simulink model "LBR7_Single_JointComputedTorque"  (R2017b)
settings: Solver=FixedStepAuto  StartTime=0.0  StopTime=12  FixedStep=0.01  RelTol=1e-3
PreLoadFcn:
  | Preload
values from neighbouring files (symbols this model uses):
  cor_gain = -1    [Preload.m]
  joint1_gain = 1    [Preload.m]    (also in PreloadTest.m)
  joint1_initial_deg = 0    [Preload.m]    (also in PreloadTest.m = 25)
  joint2_gain = 1    [Preload.m]    (also in PreloadTest.m)
  joint2_initial_deg = 0    [Preload.m]    (also in PreloadTest.m = 70)
  joint3_gain = 1    [Preload.m]    (also in PreloadTest.m)
  joint3_initial_deg = -25    [Preload.m]    (also in PreloadTest.m = 60)
  joint4_gain = 1    [Preload.m]    (also in PreloadTest.m)
  joint4_initial_deg = 90    [Preload.m]    (also in PreloadTest.m = 20)
  joint5_gain = 1    [Preload.m]    (also in PreloadTest.m)
  joint5_initial_deg = 0    [Preload.m]    (also in PreloadTest.m = 22)
  joint6_gain = 1    [Preload.m]    (also in PreloadTest.m)
  joint6_initial_deg = 90    [Preload.m]    (also in PreloadTest.m = 60)
  joint7_gain = 1    [Preload.m]    (also in PreloadTest.m)
  joint7_initial_deg = 0    [Preload.m]    (also in PreloadTest.m = 30)
  kuk = SerialLink(L)    [Preload.m]    (also in PreloadTest.m)
undefined symbols (not defined in the file or in its folder): cory, gravy, inert, X, Y, Z
libraries: sm_lib x77, nesl_utility x30
(part 1 of 3)
settings Model: Creator=jrv  LastModifiedBy=mkiri

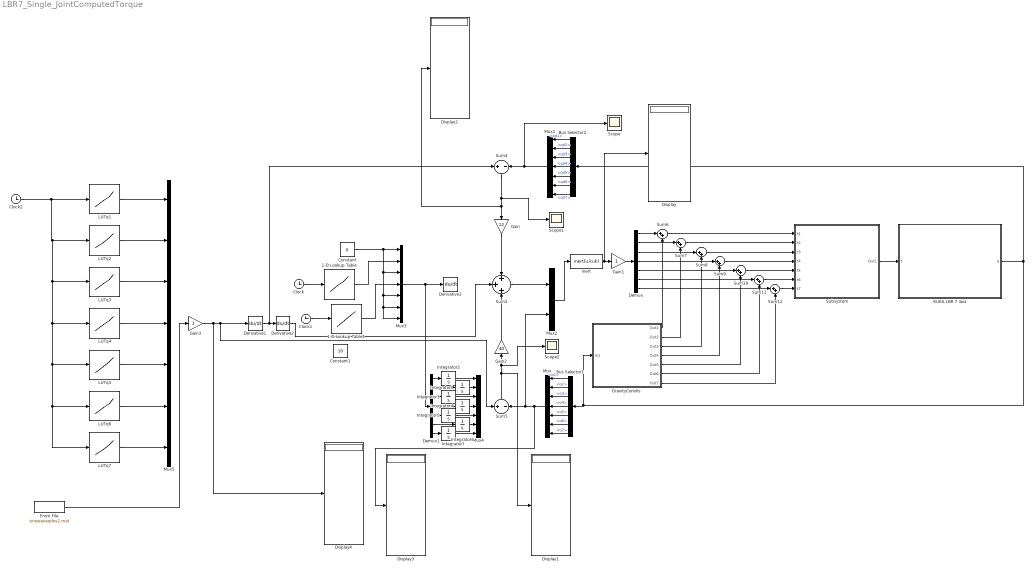
== system LBR7_Single_JointComputedTorque ==
  1-D Lookup Table : Lookup_n-D  NumberOfTableDimensions=1  BreakpointsForDimension1=[0 3 6]  Table=[0 -0.05 -0.1]  ExtrapMethod=Clip  UseLastTableValue=on  InternalRulePriority=Speed  RndMeth=Simplest  InputSameDT=on
  1-D Lookup Table1 : Lookup_n-D  NumberOfTableDimensions=1  BreakpointsForDimension1=[0 3 6]  Table=[0 -0.05 -0.1]  ExtrapMethod=Clip  UseLastTableValue=on  InternalRulePriority=Speed  RndMeth=Simplest  InputSameDT=on
  Bus Selector1 : BusSelector  OutputSignals=q1,q2,q3,q4,q5,q6,q7
  Bus Selector2 : BusSelector  OutputSignals=qd1,qd2,qd3,qd4,qd5,qd6,qd7
  Clock : Clock
  Clock1 : Clock
  Clock2 : Clock
  Constant : Constant  Value=0
  Constant1 : Constant  Value=10
  Demux : Demux  Outputs=7
  Demux1 : Demux  Outputs=7
  Derivative1 : Derivative
  Derivative2 : Derivative
  Derivative3 : Derivative
  Display{,1..4} (5 alike) : Display
  From File : FromFile  FileName=sinewaveqdes2.mat  SampleTime=0
  Gain : Gain  Gain=12
  Gain1 : Gain
  Gain2 : Gain  Gain=40
  Gain3 : Gain
  GravityCoriolis : Subsystem
  Integrator1 : Integrator  InitialCondition=joint2_initial_deg*pi/180
  Integrator2 : Integrator  InitialCondition=joint1_initial_deg*pi/180
  Integrator3 : Integrator  InitialCondition=joint3_initial_deg*pi/180
  Integrator4 : Integrator  InitialCondition=joint4_initial_deg*pi/180
  Integrator5 : Integrator  InitialCondition=joint5_initial_deg*pi/180
  Integrator6 : Integrator  InitialCondition=joint6_initial_deg*pi/180
  Integrator7 : Integrator  InitialCondition=joint7_initial_deg*pi/180
  KUKA LBR 7 iiwa : Subsystem
  LUTq1 : Lookup_n-D  NumberOfTableDimensions=1  BreakpointsForDimension1=|  Table=|  ExtrapMethod=Clip  UseLastTableValue=on  InternalRulePriority=Speed  RndMeth=Simplest  InputSameDT=on
      | [0
      | 0.1
      | 0.2
      | 0.3
      | 0.4
      | 0.5
      | 0.6
      | 0.7
      | 0.8
      | 0.9
      | 1
      | 1.1
      | 1.2
      | 1.3
      | 1.4
      | 1.5
      | 1.6
      | 1.7
      | 1.8
      | 1.9
      | 2
      | 2.1
      | 2.2
      | 2.3
      | 2.4
      | 2.5
      | 2.6
      | 2.7
      | 2.8
      | 2.9
      | 3
      | 3.1
      | 3.2
      | 3.3
      | 3.4
      | 3.5
      | 3.6
      | 3.7
      | 3.8
      | 3.9
      | 4
      | 4.1
      | 4.2
      | 4.3
      | 4.4
      | 4.5
      | 4.6
      | 4.7
      | 4.8
      | 4.9
      | 5
      | 5.1
      | 5.2
      | 5.3
      | 5.4
      | 5.5
      | 5.6
      | 5.7
      | 5.8
      | 5.9
      | 6
      | 6.1
      | 6.2
      | 6.3
      | 6.4
      | 6.5
      | 6.6
      | 6.7
      | 6.8
      | 6.9
      | 7
      | 7.1
      | 7.2
      | 7.3
      | 7.4
      | 7.5
      | 7.6
      | 7.7
      | 7.8
      | 7.9
      | 8
      | 8.1
      | 8.2
      | 8.3
      | 8.4
      | 8.5
      | 8.6
      | 8.7
      | 8.8
      | 8.9
      | 9
      | 9.1
      | 9.2
      | 9.3
      | 9.4
      | 9.5
      | 9.6
      | 9.7
      | 9.8
      | 9.9
      | 10
      | 10.1
      | 10.2
      | 10.3
      | 10.4
      | 10.5
      | 10.6
      | 10.7
      | 10.8
      | 10.9
      | 11
      | 11.1
      | 11.2
      | 11.3
      | 11.4
      | 11.5
      | 11.6
      | 11.7
      | 11.8
      | 11.9
      | 12]
      | [0
      | -0.119745838
      | -0.18133285
      | -0.22208651
      | -0.249966667
      | -0.268387869
      | -0.279374076
      | -0.2843815
      | -0.28458052
      | -0.280964237
      | -0.274392351
      | -0.265610064
      | -0.255258118
      | -0.243880509
      | -0.231932258
      | -0.219787814
      | -0.207749985
      | -0.196059015
      | -0.184901487
      | -0.17441876
      | -0.164714747
      | -0.155862933
      | -0.147912579
      | -0.140894125
      | -0.134823823
      | -0.129707667
      | -0.125544697
      | -0.122329759
      | -0.120055811
      | -0.118715875
      | -0.118304705
      | -0.118819748
      | -0.12025698
      | -0.122607535
      | -0.125859698
      | -0.13000098
      | -0.135019771
      | -0.140906638
      | -0.147655292
      | -0.155263272
      | -0.163732363
      | -0.173068797
      | -0.183283237
      | -0.194390568
      | -0.206409516
      | -0.219362074
      | -0.233272744
      | -0.248167558
      | -0.264072847
      | -0.281013701
      | -0.299012051
      | -0.318084282
      | -0.338238276
      | -0.359469746
      | -0.381757752
      | -0.405059235
      | -0.42930248
      | -0.454379451
      | -0.480137074
      | -0.506367799
      | -0.532800106
      | -0.559092165
      | -0.584849644
      | -0.609653933
      | -0.633079009
      | -0.65471118
      | -0.674171717
      | -0.691139691
      | -0.705371922
      | -0.716717459
      | -0.725125039
      | -0.730643235
      | -0.733413853
      | -0.733659638
      | -0.731667534
      | -0.727768976
      | -0.722319017
      | -0.715676313
      | -0.708185875
      | -0.700165951
      | -0.691899594
      | -0.683630649
      | -0.675563349
      | -0.667864462
      | -0.660666979
      | -0.654074526
      | -0.648165916
      | -0.642999499
      | -0.638617115
      | -0.635047627
      | -0.632310016
      | -0.630415481
      | -0.629363254
      | -0.629138645
      | -0.629717937
      | -0.631072659
      | -0.633172809
      | -0.635989263
      | -0.639495582
      | -0.64366931
      | -0.648492881
      | -0.653954144
      | -0.660046536
      | -0.666768854
      | -0.674124557
      | -0.682120437
      | -0.690764415
      | -0.700062001
      | -0.710010688
      | -0.720590981
      | -0.73175193
      | -0.743387592
      | -0.755298981
      | -0.767134702
      | -0.778307549
      | -0.787908711
      | -0.794710012
      | -0.797428487
      | -0.795301834
      | -0.788546355
      | -0.778182809]
  LUTq2 : Lookup_n-D  NumberOfTableDimensions=1  BreakpointsForDimension1=|  Table=|  ExtrapMethod=Clip  UseLastTableValue=on  InternalRulePriority=Speed  RndMeth=Simplest  InputSameDT=on
      | [0
      | 0.1
      | 0.2
      | 0.3
      | 0.4
      | 0.5
      | 0.6
      | 0.7
      | 0.8
      | 0.9
      | 1
      | 1.1
      | 1.2
      | 1.3
      | 1.4
      | 1.5
      | 1.6
      | 1.7
      | 1.8
      | 1.9
      | 2
      | 2.1
      | 2.2
      | 2.3
      | 2.4
      | 2.5
      | 2.6
      | 2.7
      | 2.8
      | 2.9
      | 3
      | 3.1
      | 3.2
      | 3.3
      | 3.4
      | 3.5
      | 3.6
      | 3.7
      | 3.8
      | 3.9
      | 4
      | 4.1
      | 4.2
      | 4.3
      | 4.4
      | 4.5
      | 4.6
      | 4.7
      | 4.8
      | 4.9
      | 5
      | 5.1
      | 5.2
      | 5.3
      | 5.4
      | 5.5
      | 5.6
      | 5.7
      | 5.8
      | 5.9
      | 6
      | 6.1
      | 6.2
      | 6.3
      | 6.4
      | 6.5
      | 6.6
      | 6.7
      | 6.8
      | 6.9
      | 7
      | 7.1
      | 7.2
      | 7.3
      | 7.4
      | 7.5
      | 7.6
      | 7.7
      | 7.8
      | 7.9
      | 8
      | 8.1
      | 8.2
      | 8.3
      | 8.4
      | 8.5
      | 8.6
      | 8.7
      | 8.8
      | 8.9
      | 9
      | 9.1
      | 9.2
      | 9.3
      | 9.4
      | 9.5
      | 9.6
      | 9.7
      | 9.8
      | 9.9
      | 10
      | 10.1
      | 10.2
      | 10.3
      | 10.4
      | 10.5
      | 10.6
      | 10.7
      | 10.8
      | 10.9
      | 11
      | 11.1
      | 11.2
      | 11.3
      | 11.4
      | 11.5
      | 11.6
      | 11.7
      | 11.8
      | 11.9
      | 12]
      | [0.4363
      | 0.550223112
      | 0.60547659
      | 0.63806274
      | 0.658275761
      | 0.670892194
      | 0.678584612
      | 0.683002774
      | 0.685224922
      | 0.685979872
      | 0.685768934
      | 0.684938338
      | 0.68372507
      | 0.682287525
      | 0.68072703
      | 0.679103595
      | 0.677447828
      | 0.67577012
      | 0.674067818
      | 0.672330815
      | 0.670545879
      | 0.668699936
      | 0.666782486
      | 0.664787266
      | 0.662713285
      | 0.660565288
      | 0.65835373
      | 0.656094298
      | 0.653807031
      | 0.65151508
      | 0.649243141
      | 0.647015831
      | 0.644857659
      | 0.642791852
      | 0.640837141
      | 0.639005272
      | 0.637299512
      | 0.635714093
      | 0.634234502
      | 0.632838482
      | 0.631497584
      | 0.630179115
      | 0.628848301
      | 0.627470531
      | 0.626013531
      | 0.624449395
      | 0.622756373
      | 0.620920382
      | 0.618936212
      | 0.616808421
      | 0.61455192
      | 0.612192264
      | 0.609765651
      | 0.607318631
      | 0.604907519
      | 0.602597483
      | 0.600461268
      | 0.598577492
      | 0.597028454
      | 0.595897398
      | 0.595265205
      | 0.595206177
      | 0.595779707
      | 0.597023358
      | 0.598951789
      | 0.601557704
      | 0.604814405
      | 0.608679693
      | 0.613100625
      | 0.618018454
      | 0.62337314
      | 0.629106939
      | 0.63516682
      | 0.641505658
      | 0.648082288
      | 0.654860655
      | 0.661808379
      | 0.668895094
      | 0.676090936
      | 0.683365433
      | 0.690686961
      | 0.698022751
      | 0.705339377
      | 0.712603584
      | 0.719783298
      | 0.726848725
      | 0.733773401
      | 0.740535164
      | 0.747116952
      | 0.753507414
      | 0.759701282
      | 0.765699535
      | 0.771509961
      | 0.777146744
      | 0.782628682
      | 0.787977284
      | 0.79321493
      | 0.798363171
      | 0.803441235
      | 0.808464774
      | 0.813444894
      | 0.818387476
      | 0.823292784
      | 0.828155308
      | 0.832963783
      | 0.837701261
      | 0.842345064
      | 0.84686637
      | 0.851229017
      | 0.855386936
      | 0.859279197
      | 0.862821119
      | 0.86588908
      | 0.868296176
      | 0.8697578
      | 0.869857026
      | 0.868049498
      | 0.863782586
      | 0.856745628
      | 0.847060856
      | 0.835195824
      | ]
  LUTq3 : Lookup_n-D  NumberOfTableDimensions=1  BreakpointsForDimension1=|  Table=|  ExtrapMethod=Clip  UseLastTableValue=on  InternalRulePriority=Speed  RndMeth=Simplest  InputSameDT=on
      | [0
      | 0.1
      | 0.2
      | 0.3
      | 0.4
      | 0.5
      | 0.6
      | 0.7
      | 0.8
      | 0.9
      | 1
      | 1.1
      | 1.2
      | 1.3
      | 1.4
      | 1.5
      | 1.6
      | 1.7
      | 1.8
      | 1.9
      | 2
      | 2.1
      | 2.2
      | 2.3
      | 2.4
      | 2.5
      | 2.6
      | 2.7
      | 2.8
      | 2.9
      | 3
      | 3.1
      | 3.2
      | 3.3
      | 3.4
      | 3.5
      | 3.6
      | 3.7
      | 3.8
      | 3.9
      | 4
      | 4.1
      | 4.2
      | 4.3
      | 4.4
      | 4.5
      | 4.6
      | 4.7
      | 4.8
      | 4.9
      | 5
      | 5.1
      | 5.2
      | 5.3
      | 5.4
      | 5.5
      | 5.6
      | 5.7
      | 5.8
      | 5.9
      | 6
      | 6.1
      | 6.2
      | 6.3
      | 6.4
      | 6.5
      | 6.6
      | 6.7
      | 6.8
      | 6.9
      | 7
      | 7.1
      | 7.2
      | 7.3
      | 7.4
      | 7.5
      | 7.6
      | 7.7
      | 7.8
      | 7.9
      | 8
      | 8.1
      | 8.2
      | 8.3
      | 8.4
      | 8.5
      | 8.6
      | 8.7
      | 8.8
      | 8.9
      | 9
      | 9.1
      | 9.2
      | 9.3
      | 9.4
      | 9.5
      | 9.6
      | 9.7
      | 9.8
      | 9.9
      | 10
      | 10.1
      | 10.2
      | 10.3
      | 10.4
      | 10.5
      | 10.6
      | 10.7
      | 10.8
      | 10.9
      | 11
      | 11.1
      | 11.2
      | 11.3
      | 11.4
      | 11.5
      | 11.6
      | 11.7
      | 11.8
      | 11.9
      | 12]
      | [-0.5236
      | -0.403227159
      | -0.366746433
      | -0.34631892
      | -0.332303097
      | -0.321933585
      | -0.314188351
      | -0.308608189
      | -0.304924638
      | -0.302925561
      | -0.302406834
      | -0.303158825
      | -0.304967031
      | -0.307617639
      | -0.310903795
      | -0.314630747
      | -0.318619272
      | -0.322707392
      | -0.326750662
      | -0.330621406
      | -0.334207281
      | -0.337409467
      | -0.340140767
      | -0.342323784
      | -0.343889307
      | -0.344774983
      | -0.344924313
      | -0.34428597
      | -0.342813423
      | -0.340464827
      | -0.337203133
      | -0.332996792
      | -0.327824919
      | -0.321681874
      | -0.31457676
      | -0.306532085
      | -0.29758211
      | -0.287770928
      | -0.277150386
      | -0.265777924
      | -0.253714417
      | -0.241022111
      | -0.227762714
      | -0.213995724
      | -0.199777023
      | -0.185157794
      | -0.170183781
      | -0.154894923
      | -0.139325364
      | -0.123503855
      | -0.107454559
      | -0.091198256
      | -0.074753954
      | -0.058140922
      | -0.041381119
      | -0.024502019
      | -0.007539775
      | 0.009457369
      | 0.026425598
      | 0.043282254
      | 0.059923224
      | 0.076222308
      | 0.092040256
      | 0.107237272
      | 0.121680738
      | 0.135253445
      | 0.147861844
      | 0.159443025
      | 0.169969282
      | 0.179449686
      | 0.187928682
      | 0.195482251
      | 0.202212424
      | 0.208240871
      | 0.213702137
      | 0.21873696
      | 0.22348605
      | 0.22808466
      | 0.232658266
      | 0.237319524
      | 0.242166487
      | 0.247281912
      | 0.252733366
      | 0.258573829
      | 0.264842496
      | 0.271565585
      | 0.278757001
      | 0.286418807
      | 0.294541475
      | 0.303103958
      | 0.312073648
      | 0.321406312
      | 0.331046609
      | 0.34093011
      | 0.350985771
      | 0.361138246
      | 0.371310047
      | 0.381423577
      | 0.391403047
      | 0.401176223
      | 0.410675983
      | 0.419841618
      | 0.428619844
      | 0.43696548
      | 0.444841759
      | 0.452220254
      | 0.459080417
      | 0.465408726
      | 0.471197447
      | 0.476443019
      | 0.481144078
      | 0.485299157
      | 0.488904235
      | 0.491950602
      | 0.494424397
      | 0.496310891
      | 0.497608556
      | 0.498355137
      | 0.498652094
      | 0.498659221
      | 0.498556154
      | ]
  LUTq4 : Lookup_n-D  NumberOfTableDimensions=1  BreakpointsForDimension1=|  Table=|  ExtrapMethod=Clip  UseLastTableValue=on  InternalRulePriority=Speed  RndMeth=Simplest  InputSameDT=on
      | [0
      | 0.1
      | 0.2
      | 0.3
      | 0.4
      | 0.5
      | 0.6
      | 0.7
      | 0.8
      | 0.9
      | 1
      | 1.1
      | 1.2
      | 1.3
      | 1.4
      | 1.5
      | 1.6
      | 1.7
      | 1.8
      | 1.9
      | 2
      | 2.1
      | 2.2
      | 2.3
      | 2.4
      | 2.5
      | 2.6
      | 2.7
      | 2.8
      | 2.9
      | 3
      | 3.1
      | 3.2
      | 3.3
      | 3.4
      | 3.5
      | 3.6
      | 3.7
      | 3.8
      | 3.9
      | 4
      | 4.1
      | 4.2
      | 4.3
      | 4.4
      | 4.5
      | 4.6
      | 4.7
      | 4.8
      | 4.9
      | 5
      | 5.1
      | 5.2
      | 5.3
      | 5.4
      | 5.5
      | 5.6
      | 5.7
      | 5.8
      | 5.9
      | 6
      | 6.1
      | 6.2
      | 6.3
      | 6.4
      | 6.5
      | 6.6
      | 6.7
      | 6.8
      | 6.9
      | 7
      | 7.1
      | 7.2
      | 7.3
      | 7.4
      | 7.5
      | 7.6
      | 7.7
      | 7.8
      | 7.9
      | 8
      | 8.1
      | 8.2
      | 8.3
      | 8.4
      | 8.5
      | 8.6
      | 8.7
      | 8.8
      | 8.9
      | 9
      | 9.1
      | 9.2
      | 9.3
      | 9.4
      | 9.5
      | 9.6
      | 9.7
      | 9.8
      | 9.9
      | 10
      | 10.1
      | 10.2
      | 10.3
      | 10.4
      | 10.5
      | 10.6
      | 10.7
      | 10.8
      | 10.9
      | 11
      | 11.1
      | 11.2
      | 11.3
      | 11.4
      | 11.5
      | 11.6
      | 11.7
      | 11.8
      | 11.9
      | 12]
      | [0.4014
      | 0.724112796
      | 0.919094054
      | 1.062533588
      | 1.175951555
      | 1.269387439
      | 1.348562596
      | 1.417113891
      | 1.477513563
      | 1.531517428
      | 1.580409811
      | 1.625149031
      | 1.666459469
      | 1.704892791
      | 1.740870318
      | 1.774713328
      | 1.806665311
      | 1.836908691
      | 1.865577623
      | 1.892767916
      | 1.918544818
      | 1.942949167
      | 1.966002263
      | 1.987709721
      | 2.008064517
      | 2.027049345
      | 2.044638435
      | 2.060798891
      | 2.075491645
      | 2.088672074
      | 2.100290343
      | 2.110292565
      | 2.11863198
      | 2.125278478
      | 2.130217032
      | 2.133445527
      | 2.134973068
      | 2.13481871
      | 2.133010555
      | 2.129585152
      | 2.124587154
      | 2.118069162
      | 2.11009171
      | 2.100723339
      | 2.090040735
      | 2.078128878
      | 2.065081209
      | 2.05099977
      | 2.035995343
      | 2.020187555
      | 2.003704964
      | 1.986685125
      | 1.96927463
      | 1.951629116
      | 1.933913244
      | 1.916300614
      | 1.898973622
      | 1.882123206
      | 1.865948478
      | 1.850656184
      | 1.836459973
      | 1.82357771
      | 1.812211787
      | 1.802530726
      | 1.79466865
      | 1.788726542
      | 1.78477359
      | 1.782848709
      | 1.782962237
      | 1.785097845
      | 1.789214631
      | 1.795249374
      | 1.803118899
      | 1.8127225
      | 1.823944359
      | 1.836655905
      | 1.85071806
      | 1.86598333
      | 1.882297708
      | 1.899502376
      | 1.917435185
      | 1.93593192
      | 1.954827367
      | 1.973956176
      | 1.993153558
      | 2.012255823
      | 2.031100783
      | 2.049528036
      | 2.067379145
      | 2.084497724
      | 2.100729435
      | 2.115923001
      | 2.129941693
      | 2.142672955
      | 2.154026248
      | 2.163930098
      | 2.172329481
      | 2.179183503
      | 2.184463354
      | 2.188150503
      | 2.190235117
      | 2.19071469
      | 2.189592848
      | 2.186878343
      | 2.182584193
      | 2.176726969
      | 2.169326212
      | 2.160403959
      | 2.149984371
      | 2.138093437
      | 2.124758752
      | 2.110009346
      | 2.093875555
      | 2.076388936
      | 2.057582191
      | 2.037489126
      | 2.016144613
      | 1.99358458
      | 1.969845992
      | 1.944966865
      | 1.918986274
      | ]
  LUTq5 : Lookup_n-D  NumberOfTableDimensions=1  BreakpointsForDimension1=|  Table=|  ExtrapMethod=Clip  UseLastTableValue=on  InternalRulePriority=Speed  RndMeth=Simplest  InputSameDT=on
      | [0
      | 0.1
      | 0.2
      | 0.3
      | 0.4
      | 0.5
      | 0.6
      | 0.7
      | 0.8
      | 0.9
      | 1
      | 1.1
      | 1.2
      | 1.3
      | 1.4
      | 1.5
      | 1.6
      | 1.7
      | 1.8
      | 1.9
      | 2
      | 2.1
      | 2.2
      | 2.3
      | 2.4
      | 2.5
      | 2.6
      | 2.7
      | 2.8
      | 2.9
      | 3
      | 3.1
      | 3.2
      | 3.3
      | 3.4
      | 3.5
      | 3.6
      | 3.7
      | 3.8
      | 3.9
      | 4
      | 4.1
      | 4.2
      | 4.3
      | 4.4
      | 4.5
      | 4.6
      | 4.7
      | 4.8
      | 4.9
      | 5
      | 5.1
      | 5.2
      | 5.3
      | 5.4
      | 5.5
      | 5.6
      | 5.7
      | 5.8
      | 5.9
      | 6
      | 6.1
      | 6.2
      | 6.3
      | 6.4
      | 6.5
      | 6.6
      | 6.7
      | 6.8
      | 6.9
      | 7
      | 7.1
      | 7.2
      | 7.3
      | 7.4
      | 7.5
      | 7.6
      | 7.7
      | 7.8
      | 7.9
      | 8
      | 8.1
      | 8.2
      | 8.3
      | 8.4
      | 8.5
      | 8.6
      | 8.7
      | 8.8
      | 8.9
      | 9
      | 9.1
      | 9.2
      | 9.3
      | 9.4
      | 9.5
      | 9.6
      | 9.7
      | 9.8
      | 9.9
      | 10
      | 10.1
      | 10.2
      | 10.3
      | 10.4
      | 10.5
      | 10.6
      | 10.7
      | 10.8
      | 10.9
      | 11
      | 11.1
      | 11.2
      | 11.3
      | 11.4
      | 11.5
      | 11.6
      | 11.7
      | 11.8
      | 11.9
      | 12]
      | [0.4014
      | 0.393329796
      | 0.433958452
      | 0.47081677
      | 0.500354569
      | 0.522694917
      | 0.538600748
      | 0.548943931
      | 0.554567179
      | 0.556239989
      | 0.554645889
      | 0.550383066
      | 0.543971154
      | 0.535860513
      | 0.526441893
      | 0.516055439
      | 0.504998544
      | 0.493532466
      | 0.481887804
      | 0.470268993
      | 0.458858
      | 0.447817388
      | 0.437292876
      | 0.427415495
      | 0.418303429
      | 0.410063583
      | 0.402792934
      | 0.396579696
      | 0.391504333
      | 0.387640446
      | 0.385055579
      | 0.383811249
      | 0.383956187
      | 0.385520489
      | 0.388517219
      | 0.392944668
      | 0.398788524
      | 0.40602396
      | 0.414617615
      | 0.424529446
      | 0.435714437
      | 0.448124132
      | 0.461707975
      | 0.476414415
      | 0.492191757
      | 0.508988712
      | 0.526754626
      | 0.545439344
      | 0.564992677
      | 0.585363446
      | 0.606498063
      | 0.628338641
      | 0.650820603
      | 0.673869794
      | 0.697399131
      | 0.721304851
      | 0.745462498
      | 0.769722905
      | 0.793908544
      | 0.817810801
      | 0.841188916
      | 0.863773014
      | 0.885286487
      | 0.905472034
      | 0.924103351
      | 0.94099445
      | 0.956006223
      | 0.96904885
      | 0.980079731
      | 0.989097981
      | 0.996137503
      | 1.001260832
      | 1.004555286
      | 1.006131713
      | 1.006124931
      | 1.004694228
      | 1.002022355
      | 0.998312095
      | 0.993780478
      | 0.988651495
      | 0.983148504
      | 0.977487431
      | 0.971871456
      | 0.96648746
      | 0.96150411
      | 0.957071313
      | 0.953320664
      | 0.950366554
      | 0.94830768
      | 0.947228787
      | 0.94720253
      | 0.948290627
      | 0.950537509
      | 0.953966505
      | 0.958584952
      | 0.964389312
      | 0.971369575
      | 0.979513106
      | 0.98880807
      | 0.99924655
      | 1.010827438
      | 1.0235592
      | 1.03746259
      | 1.052573404
      | 1.068945391
      | 1.08665344
      | 1.105797191
      | 1.126505179
      | 1.148939577
      | 1.173301308
      | 1.199834678
      | 1.228829071
      | 1.260611612
      | 1.295516955
      | 1.333806502
      | 1.375494802
      | 1.420064907
      | 1.466207368
      | 1.511954808
      | 1.55538916
      | 1.595349716
      | ]
  LUTq6 : Lookup_n-D  NumberOfTableDimensions=1  BreakpointsForDimension1=|  Table=|  ExtrapMethod=Clip  UseLastTableValue=on  InternalRulePriority=Speed  RndMeth=Simplest  InputSameDT=on
      | [0
      | 0.1
      | 0.2
      | 0.3
      | 0.4
      | 0.5
      | 0.6
      | 0.7
      | 0.8
      | 0.9
      | 1
      | 1.1
      | 1.2
      | 1.3
      | 1.4
      | 1.5
      | 1.6
      | 1.7
      | 1.8
      | 1.9
      | 2
      | 2.1
      | 2.2
      | 2.3
      | 2.4
      | 2.5
      | 2.6
      | 2.7
      | 2.8
      | 2.9
      | 3
      | 3.1
      | 3.2
      | 3.3
      | 3.4
      | 3.5
      | 3.6
      | 3.7
      | 3.8
      | 3.9
      | 4
      | 4.1
      | 4.2
      | 4.3
      | 4.4
      | 4.5
      | 4.6
      | 4.7
      | 4.8
      | 4.9
      | 5
      | 5.1
      | 5.2
      | 5.3
      | 5.4
      | 5.5
      | 5.6
      | 5.7
      | 5.8
      | 5.9
      | 6
      | 6.1
      | 6.2
      | 6.3
      | 6.4
      | 6.5
      | 6.6
      | 6.7
      | 6.8
      | 6.9
      | 7
      | 7.1
      | 7.2
      | 7.3
      | 7.4
      | 7.5
      | 7.6
      | 7.7
      | 7.8
      | 7.9
      | 8
      | 8.1
      | 8.2
      | 8.3
      | 8.4
      | 8.5
      | 8.6
      | 8.7
      | 8.8
      | 8.9
      | 9
      | 9.1
      | 9.2
      | 9.3
      | 9.4
      | 9.5
      | 9.6
      | 9.7
      | 9.8
      | 9.9
      | 10
      | 10.1
      | 10.2
      | 10.3
      | 10.4
      | 10.5
      | 10.6
      | 10.7
      | 10.8
      | 10.9
      | 11
      | 11.1
      | 11.2
      | 11.3
      | 11.4
      | 11.5
      | 11.6
      | 11.7
      | 11.8
      | 11.9
      | 12]
      | [0.1571
      | 0.242859047
      | 0.271770787
      | 0.281988745
      | 0.284065472
      | 0.282702722
      | 0.280361558
      | 0.278404652
      | 0.277581854
      | 0.278277778
      | 0.280653307
      | 0.284731849
      | 0.290453455
      | 0.297708976
      | 0.306361422
      | 0.316259066
      | 0.32724325
      | 0.339152845
      | 0.351826654
      | 0.365104565
      | 0.378828004
      | 0.392840002
      | 0.406985096
      | 0.421109183
      | 0.435059402
      | 0.448684106
      | 0.461832929
      | 0.474356985
      | 0.486109192
      | 0.496944722
      | 0.50672157
      | 0.515302177
      | 0.522564434
      | 0.528411767
      | 0.532773074
      | 0.535601542
      | 0.536873244
      | 0.53658548
      | 0.534754873
      | 0.53141526
      | 0.526615423
      | 0.520416762
      | 0.512890962
      | 0.50411775
      | 0.494182819
      | 0.483175958
      | 0.47118945
      | 0.458316771
      | 0.444651599
      | 0.430287161
      | 0.415315919
      | 0.399829616
      | 0.383919693
      | 0.367678129
      | 0.351198733
      | 0.334578984
      | 0.317922508
      | 0.301342284
      | 0.284964684
      | 0.268934348
      | 0.253419792
      | 0.238617693
      | 0.224739924
      | 0.211997744
      | 0.200599075
      | 0.190744219
      | 0.182618772
      | 0.176384714
      | 0.172171106
      | 0.170065882
      | 0.17010995
      | 0.172294318
      | 0.176560485
      | 0.182804022
      | 0.190880989
      | 0.200616584
      | 0.211815094
      | 0.224270019
      | 0.237773191
      | 0.252122001
      | 0.267124272
      | 0.282600797
      | 0.298385888
      | 0.314326477
      | 0.330280289
      | 0.346113541
      | 0.361698504
      | 0.376911147
      | 0.39162899
      | 0.405729253
      | 0.419087328
      | 0.43157664
      | 0.443078754
      | 0.453492301
      | 0.462731549
      | 0.470724678
      | 0.477412647
      | 0.482748448
      | 0.486696622
      | 0.489232906
      | 0.49034393
      | 0.490026934
      | 0.488289484
      | 0.485149242
      | 0.48063388
      | 0.474781336
      | 0.467640686
      | 0.459274143
      | 0.449760941
      | 0.439204386
      | 0.427744184
      | 0.415577441
      | 0.402993515
      | 0.3904291
      | 0.378545956
      | 0.368310527
      | 0.360989475
      | 0.357895963
      | 0.359840952
      | 0.366695844
      | 0.377555344
      | ]
  LUTq7 : Lookup_n-D  NumberOfTableDimensions=1  BreakpointsForDimension1=|  Table=|  ExtrapMethod=Clip  UseLastTableValue=on  InternalRulePriority=Speed  RndMeth=Simplest  InputSameDT=on
      | [0
      | 0.1
      | 0.2
      | 0.3
      | 0.4
      | 0.5
      | 0.6
      | 0.7
      | 0.8
      | 0.9
      | 1
      | 1.1
      | 1.2
      | 1.3
      | 1.4
      | 1.5
      | 1.6
      | 1.7
      | 1.8
      | 1.9
      | 2
      | 2.1
      | 2.2
      | 2.3
      | 2.4
      | 2.5
      | 2.6
      | 2.7
      | 2.8
      | 2.9
      | 3
      | 3.1
      | 3.2
      | 3.3
      | 3.4
      | 3.5
      | 3.6
      | 3.7
      | 3.8
      | 3.9
      | 4
      | 4.1
      | 4.2
      | 4.3
      | 4.4
      | 4.5
      | 4.6
      | 4.7
      | 4.8
      | 4.9
      | 5
      | 5.1
      | 5.2
      | 5.3
      | 5.4
      | 5.5
      | 5.6
      | 5.7
      | 5.8
      | 5.9
      | 6
      | 6.1
      | 6.2
      | 6.3
      | 6.4
      | 6.5
      | 6.6
      | 6.7
      | 6.8
      | 6.9
      | 7
      | 7.1
      | 7.2
      | 7.3
      | 7.4
      | 7.5
      | 7.6
      | 7.7
      | 7.8
      | 7.9
      | 8
      | 8.1
      | 8.2
      | 8.3
      | 8.4
      | 8.5
      | 8.6
      | 8.7
      | 8.8
      | 8.9
      | 9
      | 9.1
      | 9.2
      | 9.3
      | 9.4
      | 9.5
      | 9.6
      | 9.7
      | 9.8
      | 9.9
      | 10
      | 10.1
      | 10.2
      | 10.3
      | 10.4
      | 10.5
      | 10.6
      | 10.7
      | 10.8
      | 10.9
      | 11
      | 11.1
      | 11.2
      | 11.3
      | 11.4
      | 11.5
      | 11.6
      | 11.7
      | 11.8
      | 11.9
      | 12]
      | [0.1396
      | 0.158447132
      | 0.160655829
      | 0.163576378
      | 0.167245985
      | 0.171195582
      | 0.175088059
      | 0.178726039
      | 0.182015187
      | 0.184932121
      | 0.187499377
      | 0.189766137
      | 0.191793753
      | 0.193645358
      | 0.19537888
      | 0.197042752
      | 0.198673642
      | 0.200295611
      | 0.201920192
      | 0.203547046
      | 0.205164899
      | 0.206752611
      | 0.20828026
      | 0.209710189
      | 0.210997989
      | 0.212093426
      | 0.212941325
      | 0.213482418
      | 0.213654177
      | 0.213391651
      | 0.212628294
      | 0.211297225
      | 0.209336718
      | 0.206695612
      | 0.203334184
      | 0.199224208
      | 0.194348673
      | 0.188701191
      | 0.182285157
      | 0.175112741
      | 0.167203777
      | 0.15858464
      | 0.149287176
      | 0.139347752
      | 0.128806484
      | 0.117706669
      | 0.106094474
      | 0.094018877
      | 0.081531884
      | 0.068689015
      | 0.055550051
      | 0.042180022
      | 0.028650397
      | 0.015040412
      | 0.001438434
      | -0.01205678
      | -0.025335171
      | -0.038275122
      | -0.050744257
      | -0.06260181
      | -0.073703026
      | -0.083906725
      | -0.093092533
      | -0.101176744
      | -0.108117362
      | -0.113914621
      | -0.118606497
      | -0.122259015
      | -0.124952606
      | -0.126767138
      | -0.127768808
      | -0.128001691
      | -0.127485548
      | -0.126219858
      | -0.124192565
      | -0.121391046
      | -0.117812608
      | -0.113472343
      | -0.108407251
      | -0.102676634
      | -0.096359636
      | -0.089551153
      | -0.082357262
      | -0.074891025
      | -0.067269132
      | -0.059609532
      | -0.05203003
      | -0.044647671
      | -0.037578759
      | -0.030939311
      | -0.024845837
      | -0.019415507
      | -0.014758615
      | -0.010971949
      | -0.00814049
      | -0.006339626
      | -0.005637095
      | -0.006094713
      | -0.007769975
      | -0.010717601
      | -0.014991126
      | -0.020644627
      | -0.027734713
      | -0.036322902
      | -0.04647856
      | -0.058282622
      | -0.071832388
      | -0.087247749
      | -0.10467933
      | -0.124319078
      | -0.146413687
      | -0.17128057
      | -0.199323609
      | -0.231039243
      | -0.266987549
      | -0.307674711
      | -0.353276636
      | -0.403233941
      | -0.456052807
      | -0.509731998
      | -0.562554297
      | ]
  Mux{,1,3..5} (5 alike) : Mux  Inputs=7
  Mux2 : Mux  Inputs=2
  Scope : Scope
  Scope1 : Scope
  Scope2 : Scope
  Subsystem : Subsystem
  Sum{6..12} (7 alike) : Sum  Inputs=|++
  Sum2 : Sum  Inputs=+++
  Sum4 : Sum  Inputs=+-
  Sum5 : Sum  Inputs=+-
  inert : MATLABFcn  MATLABFcn=inert(u,kuk)
  wires:
  Subsystem/1(Out1) -> KUKA LBR 7 iiwa/1(t)
  Bus Selector1/5 -> Mux/5  "<q5>"
  Bus Selector1/3 -> Mux/3  "<q3>"
  Bus Selector1/7 -> Mux/7  "<q7>"
  Bus Selector1/6 -> Mux/6  "<q6>"
  Bus Selector1/2 -> Mux/2  "<q2>"
  Bus Selector1/4 -> Mux/4  "<q4>"
  Bus Selector2/5 -> Mux1/5  "<qd5>"
  Bus Selector2/4 -> Mux1/4  "<qd4>"
  Bus Selector2/3 -> Mux1/3  "<qd3>"
  Bus Selector2/2 -> Mux1/2  "<qd2>"
  Bus Selector2/1 -> Mux1/1  "<qd1>"
  Mux3/1 -> Demux1/1, Derivative3/1
  Mux1/1 -> Scope/1, Sum4/2
  Bus Selector2/6 -> Mux1/6  "<qd6>"
  KUKA LBR 7 iiwa/1(q) -> Bus Selector1/1, GravityCoriolis/1(In1), Bus Selector2/1
  Bus Selector2/7 -> Mux1/7  "<qd7>"
  Sum4/1 -> Scope1/1, Display2/1, Gain/1
  Sum5/1 -> Display1/1, Scope2/1, Gain2/1
  Mux/1 -> Display3/1, Mux2/2, Sum5/2
  Mux2/1 -> inert/1
  GravityCoriolis/1(Out1) -> Sum6/2
  Sum8/1 -> Subsystem/3(t3)
  GravityCoriolis/4(Out4) -> Sum9/2
  GravityCoriolis/2(Out2) -> Sum7/2
  Sum9/1 -> Subsystem/4(t4)
  Sum11/1 -> Subsystem/6(t6)
  Demux/7 -> Sum12/1
  Demux/5 -> Sum10/1
  GravityCoriolis/5(Out5) -> Sum10/2
  Sum6/1 -> Subsystem/1(t1)
  Demux/1 -> Sum6/1
  inert/1 -> Display/1, Gain1/1
  Sum10/1 -> Subsystem/5(t5)
  Demux/6 -> Sum11/1
  Demux/3 -> Sum8/1
  GravityCoriolis/6(Out6) -> Sum11/2
  Demux/4 -> Sum9/1
  Demux/2 -> Sum7/1
  Sum7/1 -> Subsystem/2(t2)
  GravityCoriolis/3(Out3) -> Sum8/2
  Sum12/1 -> Subsystem/7(t7)
  GravityCoriolis/7(Out7) -> Sum12/2
  Bus Selector1/1 -> Mux/1  "<q1>"
  Clock/1 -> 1-D Lookup Table/1
  Constant/1 -> Mux3/5, Mux3/6, Mux3/7, Mux3/3, Mux3/1
  Gain1/1 -> Demux/1
  Demux1/1 -> Integrator2/1
  Demux1/2 -> Integrator1/1
  Demux1/3 -> Integrator3/1
  Demux1/4 -> Integrator4/1
  Demux1/5 -> Integrator5/1
  Demux1/6 -> Integrator6/1
  Demux1/7 -> Integrator7/1
  1-D Lookup Table/1 -> Mux3/2
  Integrator1/1 -> Mux4/2
  Integrator2/1 -> Mux4/1
  Integrator3/1 -> Mux4/3
  Integrator4/1 -> Mux4/4
  Integrator5/1 -> Mux4/5
  Integrator6/1 -> Mux4/6
  Integrator7/1 -> Mux4/7
  Sum2/1 -> Mux2/1
  Gain/1 -> Sum2/1
  Gain2/1 -> Sum2/3
  Clock1/1 -> 1-D Lookup Table1/1
  1-D Lookup Table1/1 -> Mux3/4
  LUTq2/1 -> Mux5/2
  LUTq3/1 -> Mux5/3
  LUTq1/1 -> Mux5/1
  LUTq4/1 -> Mux5/4
  LUTq5/1 -> Mux5/5
  LUTq6/1 -> Mux5/6
  LUTq7/1 -> Mux5/7
  Derivative1/1 -> Sum4/1, Derivative2/1
  Derivative2/1 -> Sum2/2
  Clock2/1 -> LUTq7/1, LUTq6/1, LUTq5/1, LUTq4/1, LUTq3/1, LUTq2/1, LUTq1/1
  Gain3/1 -> Display4/1, Sum5/1, Derivative1/1
  From File/1 -> Gain3/1

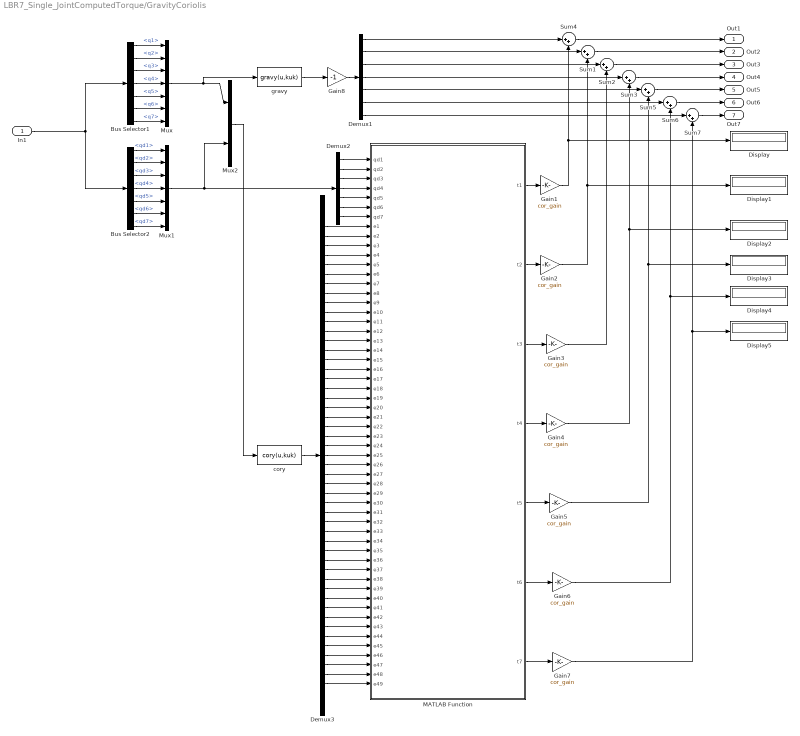
== system LBR7_Single_JointComputedTorque/GravityCoriolis ==
  In1 : Inport
  Bus Selector1 : BusSelector  OutputSignals=q1,q2,q3,q4,q5,q6,q7
  Bus Selector2 : BusSelector  OutputSignals=qd1,qd2,qd3,qd4,qd5,qd6,qd7
  Demux1 : Demux  Outputs=7
  Demux2 : Demux  Outputs=7
  Demux3 : Demux  Outputs=49
  Display{,1..5} (6 alike) : Display
  Gain{1..7} (7 alike) : Gain  Gain=cor_gain
  Gain8 : Gain  Gain=-1
  MATLAB Function : MATLAB Function  TreatAsAtomicUnit=on
  Mux : Mux  Inputs=7
  Mux1 : Mux  Inputs=7
  Mux2 : Mux  Inputs=2
  Sum{1..7} (7 alike) : Sum  Inputs=|++
  cory : MATLABFcn  MATLABFcn=cory(u,kuk)
  gravy : MATLABFcn  MATLABFcn=gravy(u,kuk)
  Out1 : Outport
  Out2 : Outport  Port=2
  Out3 : Outport  Port=3
  Out4 : Outport  Port=4
  Out5 : Outport  Port=5
  Out6 : Outport  Port=6
  Out7 : Outport  Port=7
  wires:
  Demux2/1 -> MATLAB Function/1(qd1)
  Mux1/1 -> Mux2/2, Demux2/1
  Demux3/16 -> MATLAB Function/23(e16)
  Mux/1 -> gravy/1, Mux2/1
  Bus Selector1/2 -> Mux/2  "<q2>"
  Demux3/29 -> MATLAB Function/36(e29)
  Demux3/35 -> MATLAB Function/42(e35)
  Demux3/15 -> MATLAB Function/22(e15)
  Demux3/22 -> MATLAB Function/29(e22)
  Demux3/9 -> MATLAB Function/16(e9)
  Bus Selector1/3 -> Mux/3  "<q3>"
  Demux3/11 -> MATLAB Function/18(e11)
  Bus Selector1/7 -> Mux/7  "<q7>"
  Demux3/42 -> MATLAB Function/49(e42)
  Demux3/43 -> MATLAB Function/50(e43)
  Bus Selector1/1 -> Mux/1  "<q1>"
  Bus Selector1/5 -> Mux/5  "<q5>"
  Demux3/24 -> MATLAB Function/31(e24)
  Bus Selector1/6 -> Mux/6  "<q6>"
  Demux3/26 -> MATLAB Function/33(e26)
  Bus Selector1/4 -> Mux/4  "<q4>"
  Demux3/14 -> MATLAB Function/21(e14)
  Demux3/19 -> MATLAB Function/26(e19)
  Demux3/4 -> MATLAB Function/11(e4)
  Bus Selector2/4 -> Mux1/4  "<qd4>"
  cory/1 -> Demux3/1
  Demux3/23 -> MATLAB Function/30(e23)
  Demux2/3 -> MATLAB Function/3(qd3)
  Demux3/31 -> MATLAB Function/38(e31)
  Demux2/4 -> MATLAB Function/4(qd4)
  Demux3/17 -> MATLAB Function/24(e17)
  Demux2/5 -> MATLAB Function/5(qd5)
  Demux3/3 -> MATLAB Function/10(e3)
  Demux3/20 -> MATLAB Function/27(e20)
  Demux3/36 -> MATLAB Function/43(e36)
  In1/1 -> Bus Selector2/1, Bus Selector1/1
  Bus Selector2/6 -> Mux1/6  "<qd6>"
  Demux3/40 -> MATLAB Function/47(e40)
  Demux3/8 -> MATLAB Function/15(e8)
  Demux3/45 -> MATLAB Function/52(e45)
  Demux3/28 -> MATLAB Function/35(e28)
  Demux3/41 -> MATLAB Function/48(e41)
  Bus Selector2/5 -> Mux1/5  "<qd5>"
  Demux3/49 -> MATLAB Function/56(e49)
  Demux3/27 -> MATLAB Function/34(e27)
  Demux3/13 -> MATLAB Function/20(e13)
  Demux3/6 -> MATLAB Function/13(e6)
  Demux3/30 -> MATLAB Function/37(e30)
  Demux2/7 -> MATLAB Function/7(qd7)
  Demux3/25 -> MATLAB Function/32(e25)
  Demux2/2 -> MATLAB Function/2(qd2)
  Demux3/5 -> MATLAB Function/12(e5)
  Bus Selector2/7 -> Mux1/7  "<qd7>"
  Demux3/7 -> MATLAB Function/14(e7)
  Bus Selector2/3 -> Mux1/3  "<qd3>"
  Mux2/1 -> cory/1
  Demux1/1 -> Sum4/1
  Demux3/1 -> MATLAB Function/8(e1)
  Demux3/33 -> MATLAB Function/40(e33)
  Demux3/12 -> MATLAB Function/19(e12)
  Bus Selector2/1 -> Mux1/1  "<qd1>"
  Demux1/4 -> Sum3/1
  Demux3/48 -> MATLAB Function/55(e48)
  Demux3/32 -> MATLAB Function/39(e32)
  Demux3/34 -> MATLAB Function/41(e34)
  Demux3/47 -> MATLAB Function/54(e47)
  Bus Selector2/2 -> Mux1/2  "<qd2>"
  Demux2/6 -> MATLAB Function/6(qd6)
  Sum7/1 -> Out7/1
  Demux3/39 -> MATLAB Function/46(e39)
  Sum3/1 -> Out4/1
  Sum6/1 -> Out6/1
  Demux1/3 -> Sum2/1
  Demux3/21 -> MATLAB Function/28(e21)
  Sum1/1 -> Out2/1
  Demux1/2 -> Sum1/1
  Sum4/1 -> Out1/1
  Demux1/5 -> Sum5/1
  Demux3/2 -> MATLAB Function/9(e2)
  Demux3/18 -> MATLAB Function/25(e18)
  Demux3/38 -> MATLAB Function/45(e38)
  Demux3/46 -> MATLAB Function/53(e46)
  Sum5/1 -> Out5/1
  Demux3/37 -> MATLAB Function/44(e37)
  Demux3/44 -> MATLAB Function/51(e44)
  Sum2/1 -> Out3/1
  Demux3/10 -> MATLAB Function/17(e10)
  Gain2/1 -> Display1/1, Sum1/2
  Gain4/1 -> Display2/1, Sum3/2
  Gain6/1 -> Display4/1, Sum6/2
  Gain3/1 -> Sum2/2
  Gain5/1 -> Display3/1, Sum5/2
  Demux1/7 -> Sum7/1
  Gain7/1 -> Display5/1, Sum7/2
  Gain8/1 -> Demux1/1
  Demux1/6 -> Sum6/1
  gravy/1 -> Gain8/1
  Gain1/1 -> Display/1, Sum4/2
  MATLAB Function/1(t1) -> Gain1/1
  MATLAB Function/2(t2) -> Gain2/1
  MATLAB Function/3(t3) -> Gain3/1
  MATLAB Function/4(t4) -> Gain4/1
  MATLAB Function/5(t5) -> Gain5/1
  MATLAB Function/6(t6) -> Gain6/1
  MATLAB Function/7(t7) -> Gain7/1
